simulink model "zad2_war2"  (R2014b)
settings: Solver=ode45  StartTime=0.0  StopTime=10.0  RelTol=1e-3
settings Model: Creator=kuba  LastModifiedBy=kuba

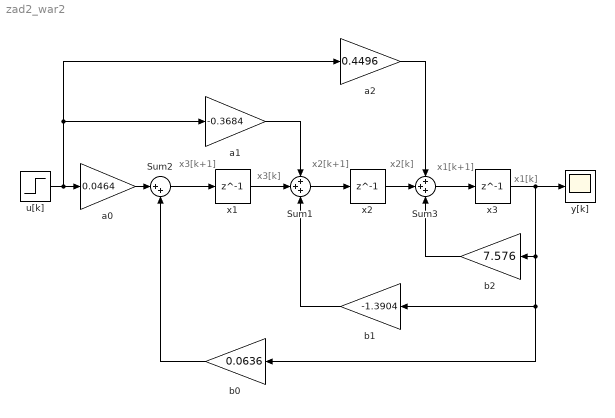
== system zad2_war2 ==
  note: x3[k]
  note: x3[k+1]
  note: x2[k]
  note: x2[k+1]
  note: x1[k]
  note: x1[k+1]
  Sum1 : Sum  Inputs=+++
  Sum2 : Sum  Inputs=|++
  Sum3 : Sum  Inputs=+++
  "a0 " : Gain  Gain=0.0464
  a1 : Gain  Gain=-0.3684
  a2 : Gain  Gain=0.4496
  "b0 " : Gain  Gain=0.0636
  b1 : Gain  Gain=-1.3904
  b2 : Gain  Gain=7.576
  u[k] : Step  SampleTime=0
  x1 : Delay  DelayLength=1
  x2 : Delay  DelayLength=1
  x3 : Delay  DelayLength=1
  y[k] : Scope
  wires:
  Sum2/1 -> x1/1
  u[k]/1 -> a2/1, a1/1, "a0 "/1
  x3/1 -> y[k]/1, "b0 "/1, b1/1, b2/1
  "a0 "/1 -> Sum2/1
  "b0 "/1 -> Sum2/2
  Sum1/1 -> x2/1
  x1/1 -> Sum1/2
  b1/1 -> Sum1/3
  a1/1 -> Sum1/1
  x2/1 -> Sum3/2
  a2/1 -> Sum3/1
  b2/1 -> Sum3/3
  Sum3/1 -> x3/1
